simulink model "Test01"  (Simulink 5.0)
settings: Solver=ode45  StartTime=0.0  StopTime=inf  FixedStep=1/100000  MaxStep=1/100000  RelTol=1e-3
libraries: commcontsrc2 x1
settings Model: LastModifiedBy=Administrator  RTWOptions="-aEnforceIntegerDowncast=1 -aExtMode=0 -aExtModeTesting=0 -aFoldNonRolledExpr=1 -aForceParamTrailComments=0 -aGenerateComments=1 -aGenerateReport=0 -aIgnoreCustomStorageClasses=1 -aIncDataTypeInIds=0 -aIncHierarchyInIds=0 -aInlineInvariantSignals=1 -aInlineParameters=0 -aInlinedPrmAccess=\"Literals\" -aLocalBlockOutputs=1 -aLogVarNameModifier=\"rt_\" -aMaxRTWIdLen=31 -aPrefixModelToSubsysFcnNames=1 -aRTWVerbose=1 -aRollThreshold=5 -aShowEliminatedStatements=0"

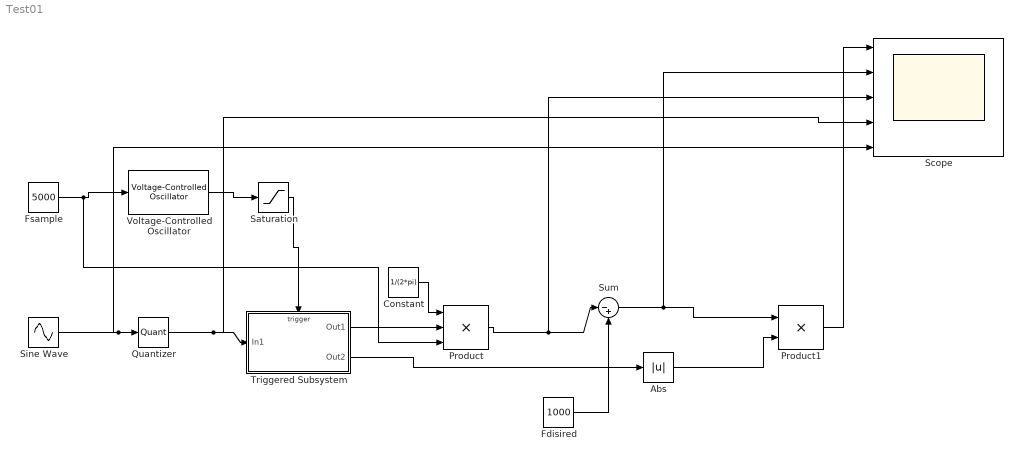
== system Test01 ==
  Abs : Abs  SaturateOnIntegerOverflow=on
  Constant : Constant  Value=1/(2*pi)
  Fdisired : Constant  Value=1000
  Fsample : Constant  Value=5000
  Product : Product  Inputs=3  SaturateOnIntegerOverflow=on
  Product1 : Product  SaturateOnIntegerOverflow=on
  Quantizer : Quantizer  QuantizationInterval=2/(2^16)
  Saturation : Saturate  UpperLimit=1  LowerLimit=-1
  Scope : Scope  NumInputPorts=5
      settings: TickLabels=on  TimeRange=0.0006  YMin=3~9.991~999.996~-1~-1  YMax=11~10.004~1000.01~1~1
  "Sine Wave " : Sin  Frequency=2*pi*1000  SampleTime=0
  Sum : Sum  Inputs=|-+  SaturateOnIntegerOverflow=on
  Triggered Subsystem : Subsystem  TreatAsAtomicUnit=on
  Voltage-Controlled Oscillator : commcontsrc2/Voltage-Controlled Oscillator  Ac=100  Fc=0  Kc=1  Ph=0
  wires:
  "Sine Wave "/1 -> Quantizer/1, Scope/5
  Quantizer/1 -> Triggered Subsystem/1(In1), Scope/4
  Saturation/1 -> Triggered Subsystem/Trigger
  Product/1 -> Sum/1, Scope/3
  Sum/1 -> Product1/1, Scope/2
  Product1/1 -> Scope/1
  Triggered Subsystem/1(Out1) -> Product/2
  Constant/1 -> Product/1
  Fdisired/1 -> Sum/2
  Triggered Subsystem/2(Out2) -> Abs/1
  Fsample/1 -> Voltage-Controlled Oscillator/1, Product/3
  Voltage-Controlled Oscillator/1 -> Saturation/1
  Abs/1 -> Product1/2

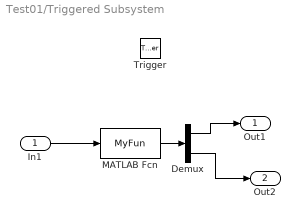
== system Test01/Triggered Subsystem ==
  In1 : Inport
  Trigger : TriggerPort
  Demux : Demux  Outputs=2
  MATLAB Fcn : MATLABFcn  MATLABFcn=MyFun  OutputDimensions=2
  Out1 : Outport
  Out2 : Outport  Port=2
  wires:
  In1/1 -> MATLAB Fcn/1
  MATLAB Fcn/1 -> Demux/1
  Demux/1 -> Out1/1
  Demux/2 -> Out2/1
